simulink model "esc_motor_model_r2017a"  (R2017a)
settings: Solver=VariableStepAuto  StartTime=0.0  StopTime=20  RelTol=1e-3
settings Model: Creator=tdarrah  LastModifiedBy=tdarrah
settings SFSimCC: SimUseLocalCustomCode=on
settings RTWCC: RTWUseLocalCustomCode=on

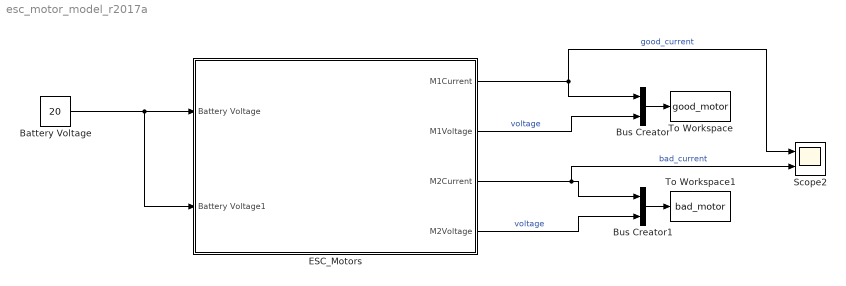
== system esc_motor_model_r2017a ==
  "Battery Voltage " : Constant  Value=20
  Bus Creator : BusCreator  Inputs=2
  Bus Creator1 : BusCreator  Inputs=2
  ESC_Motors : Subsystem
  Scope2 : Scope  NumInputPorts=2
  To Workspace : ToWorkspace  VariableName=good_motor  SaveFormat=Timeseries  SampleTime=-1
  To Workspace1 : ToWorkspace  VariableName=bad_motor  SaveFormat=Timeseries  SampleTime=-1
  wires:
  "Battery Voltage "/1 -> ESC_Motors/2(Battery Voltage1), ESC_Motors/1(Battery Voltage)
  ESC_Motors/1(M1Current) -> Scope2/1, Bus Creator/1  "good_current"
  ESC_Motors/2(M1Voltage) -> Bus Creator/2  "voltage"
  Bus Creator/1 -> To Workspace/1
  ESC_Motors/4(M2Voltage) -> Bus Creator1/2  "voltage"
  ESC_Motors/3(M2Current) -> Scope2/2, Bus Creator1/1  "bad_current"
  Bus Creator1/1 -> To Workspace1/1

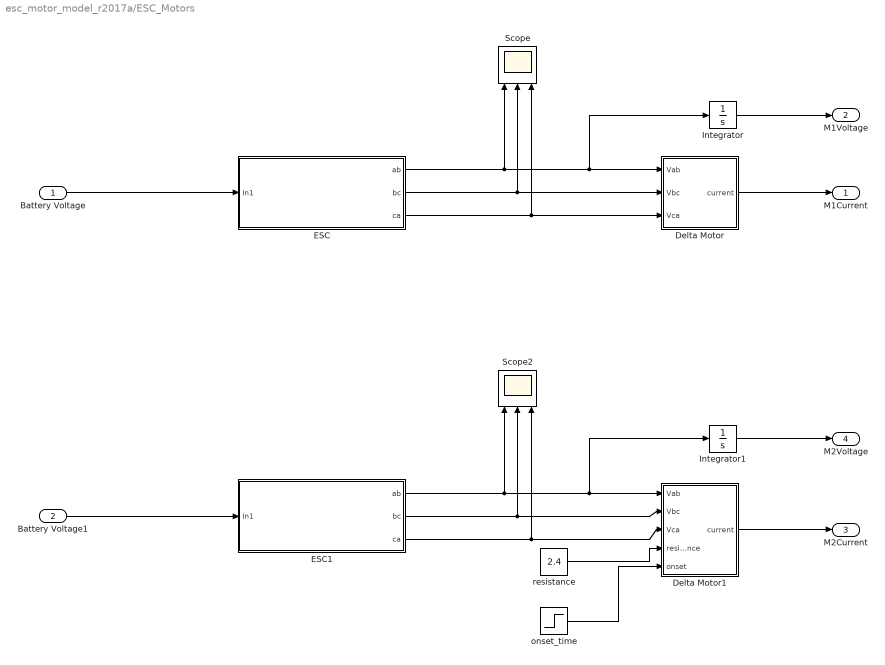
== system esc_motor_model_r2017a/ESC_Motors ==
  Battery Voltage : Inport
  Battery Voltage1 : Inport  Port=2
  Delta Motor : Subsystem
  Delta Motor1 : Subsystem
  ESC : Subsystem
  ESC1 : Subsystem
  Integrator : Integrator
  Integrator1 : Integrator
  Scope : Scope  NumInputPorts=3
  Scope2 : Scope  NumInputPorts=3
  "onset_time " : Step  Time=10  SampleTime=0
  resistance : Constant  Value=2.4
  M1Current : Outport
  M1Voltage : Outport  Port=2
  M2Current : Outport  Port=3
  M2Voltage : Outport  Port=4
  wires:
  Delta Motor/1(current) -> M1Current/1
  Integrator/1 -> M1Voltage/1
  ESC/2(bc) -> Scope/2, Delta Motor/2(Vbc)
  ESC/1(ab) -> Integrator/1, Delta Motor/1(Vab), Scope/1
  ESC/3(ca) -> Scope/3, Delta Motor/3(Vca)
  Battery Voltage/1 -> ESC/1(In1)
  Battery Voltage1/1 -> ESC1/1(In1)
  ESC1/1(ab) -> Integrator1/1, Delta Motor1/1(Vab), Scope2/1
  Delta Motor1/1(current) -> M2Current/1
  Integrator1/1 -> M2Voltage/1
  ESC1/3(ca) -> Scope2/3, Delta Motor1/3(Vca)
  ESC1/2(bc) -> Scope2/2, Delta Motor1/2(Vbc)
  resistance/1 -> Delta Motor1/4(resistance)
  "onset_time "/1 -> Delta Motor1/5(onset)

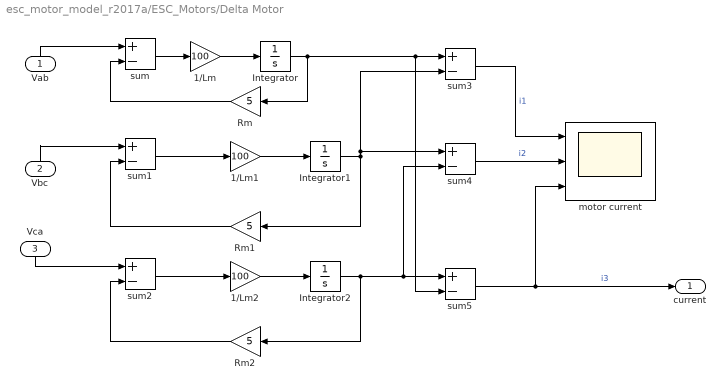
== system esc_motor_model_r2017a/ESC_Motors/Delta Motor ==
  Vab : Inport
  Vbc : Inport  Port=2
  Vca : Inport  Port=3
  1/Lm : Gain  Gain=100
  1/Lm1 : Gain  Gain=100
  1/Lm2 : Gain  Gain=100
  Integrator : Integrator
  Integrator1 : Integrator
  Integrator2 : Integrator
  Rm : Gain  Gain=5
  Rm1 : Gain  Gain=5
  Rm2 : Gain  Gain=5
  motor current : Scope  NumInputPorts=3
  sum{,1..5} (6 alike) : Sum  Inputs=+-
  current : Outport
  wires:
  1/Lm2/1 -> Integrator2/1
  Integrator/1 -> sum5/2, sum3/1, Rm/1
  sum3/1 -> motor current/1  "i1"
  Vab/1 -> sum/1
  Rm/1 -> sum/2
  Integrator1/1 -> sum4/1, sum3/2, Rm1/1
  sum1/1 -> 1/Lm1/1
  sum/1 -> 1/Lm/1
  1/Lm1/1 -> Integrator1/1
  Integrator2/1 -> sum5/1, sum4/2, Rm2/1
  1/Lm/1 -> Integrator/1
  sum4/1 -> motor current/2  "i2"
  Rm1/1 -> sum1/2
  Vca/1 -> sum2/1
  sum5/1 -> motor current/3, current/1  "i3"
  sum2/1 -> 1/Lm2/1
  Rm2/1 -> sum2/2
  Vbc/1 -> sum1/1

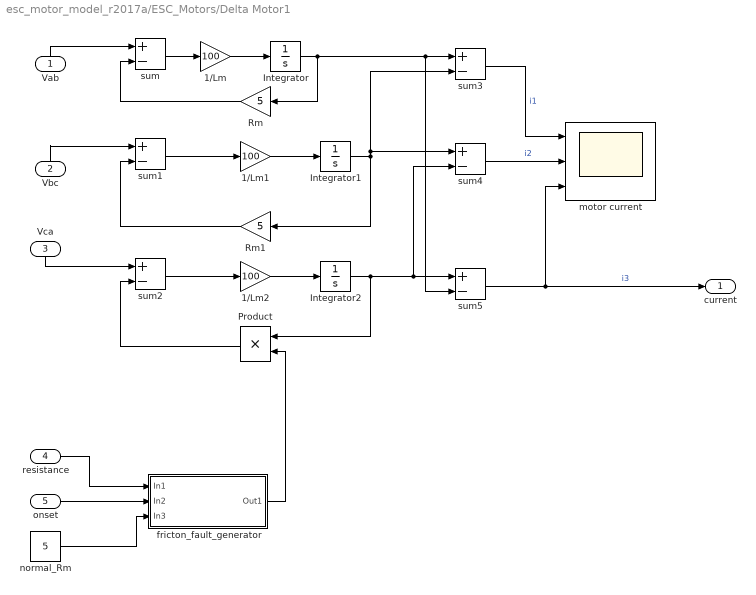
== system esc_motor_model_r2017a/ESC_Motors/Delta Motor1 ==
  Vab : Inport
  Vbc : Inport  Port=2
  Vca : Inport  Port=3
  resistance : Inport  Port=4
  onset : Inport  Port=5
  1/Lm : Gain  Gain=100
  1/Lm1 : Gain  Gain=100
  1/Lm2 : Gain  Gain=100
  Integrator : Integrator
  Integrator1 : Integrator
  Integrator2 : Integrator
  Product : Product
  Rm : Gain  Gain=5
  Rm1 : Gain  Gain=5
  fricton_fault_generator : Subsystem
  motor current : Scope  NumInputPorts=3
  normal_Rm : Constant  Value=5
  sum{,1..5} (6 alike) : Sum  Inputs=+-
  current : Outport
  wires:
  1/Lm2/1 -> Integrator2/1
  Integrator/1 -> sum5/2, sum3/1, Rm/1
  sum3/1 -> motor current/1  "i1"
  Vab/1 -> sum/1
  Rm/1 -> sum/2
  Integrator1/1 -> sum4/1, sum3/2, Rm1/1
  sum1/1 -> 1/Lm1/1
  sum/1 -> 1/Lm/1
  1/Lm1/1 -> Integrator1/1
  Integrator2/1 -> Product/1, sum5/1, sum4/2
  1/Lm/1 -> Integrator/1
  sum4/1 -> motor current/2  "i2"
  Rm1/1 -> sum1/2
  Vca/1 -> sum2/1
  sum5/1 -> motor current/3, current/1  "i3"
  sum2/1 -> 1/Lm2/1
  Product/1 -> sum2/2
  Vbc/1 -> sum1/1
  resistance/1 -> fricton_fault_generator/1(In1)
  onset/1 -> fricton_fault_generator/2(In2)
  normal_Rm/1 -> fricton_fault_generator/3(In3)
  fricton_fault_generator/1(Out1) -> Product/2

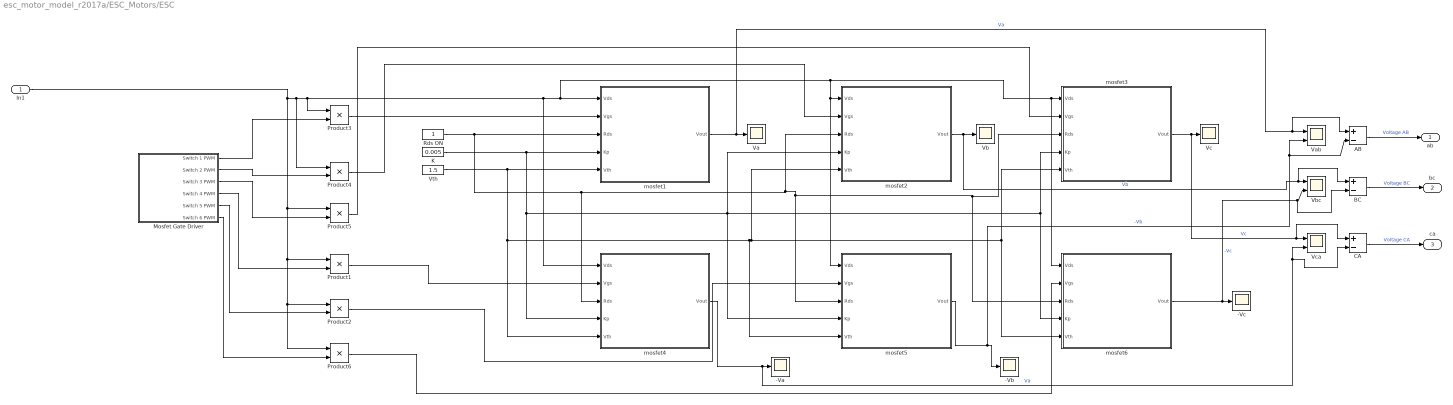
== system esc_motor_model_r2017a/ESC_Motors/ESC ==
  In1 : Inport
  -Va : Scope
  -Vb : Scope
  -Vc : Scope
  AB : Sum  Inputs=+-
  BC : Sum  Inputs=+-
  CA : Sum  Inputs=+-
  K : Constant  Value=0.005
  Mosfet Gate Driver : Subsystem
  Product{1..6} (6 alike) : Product
  Rds ON : Constant
  Va : Scope
  Vab : Scope  NumInputPorts=2
  Vb : Scope
  Vbc : Scope  NumInputPorts=2
  Vc : Scope
  Vca : Scope  NumInputPorts=2
  Vth : Constant  Value=1.5
  mosfet1 : MATLAB Function  TreatAsAtomicUnit=on
  mosfet2 : MATLAB Function  TreatAsAtomicUnit=on
  mosfet3 : MATLAB Function  TreatAsAtomicUnit=on
  mosfet4 : MATLAB Function  TreatAsAtomicUnit=on
  mosfet5 : MATLAB Function  TreatAsAtomicUnit=on
  mosfet6 : MATLAB Function  TreatAsAtomicUnit=on
  ab : Outport
  bc : Outport  Port=2
  ca : Outport  Port=3
  wires:
  mosfet2/1(Vout) -> BC/1, Vbc/1, Vb/1  "Vb"
  Mosfet Gate Driver/4(Switch 4 PWM) -> Product1/2
  CA/1 -> ca/1  "Voltage CA"
  Product5/1 -> mosfet3/2(Vgs)
  Mosfet Gate Driver/6(Switch 6 PWM) -> Product6/2
  BC/1 -> bc/1  "Voltage BC"
  Product2/1 -> mosfet5/2(Vgs)
  mosfet5/1(Vout) -> AB/2, Vab/2, -Vb/1  "-Vb"
  mosfet4/1(Vout) -> CA/2, Vca/2, -Va/1  "Va"
  Product4/1 -> mosfet2/2(Vgs)
  In1/1 -> Product6/1, Product2/1, Product1/1, Product5/1, Product4/1, mosfet4/1(Vds), mosfet6/1(Vds), mosfet3/1(Vds), mosfet5/1(Vds), mosfet2/1(Vds), mosfet1/1(Vds), Product3/1
  Mosfet Gate Driver/1(Switch 1 PWM) -> Product3/2
  mosfet6/1(Vout) -> BC/2, Vbc/2, -Vc/1  "-Vc"
  Product1/1 -> mosfet4/2(Vgs)
  AB/1 -> ab/1  "Voltage AB"
  Rds ON/1 -> mosfet1/3(Rds), mosfet4/3(Rds), mosfet3/3(Rds), mosfet6/3(Rds), mosfet5/3(Rds), mosfet2/3(Rds)
  Vth/1 -> mosfet4/5(Vth), mosfet5/5(Vth), mosfet2/5(Vth), mosfet6/5(Vth), mosfet3/5(Vth), mosfet1/5(Vth)
  mosfet3/1(Vout) -> CA/1, Vca/1, Vc/1  "Vc"
  Mosfet Gate Driver/2(Switch 2 PWM) -> Product4/2
  Mosfet Gate Driver/5(Switch 5 PWM) -> Product2/2
  Mosfet Gate Driver/3(Switch 3 PWM) -> Product5/2
  mosfet1/1(Vout) -> AB/1, Vab/1, Va/1  "Va"
  Product3/1 -> mosfet1/2(Vgs)
  K/1 -> mosfet4/4(Kp), mosfet5/4(Kp), mosfet2/4(Kp), mosfet6/4(Kp), mosfet3/4(Kp), mosfet1/4(Kp)
  Product6/1 -> mosfet6/2(Vgs)

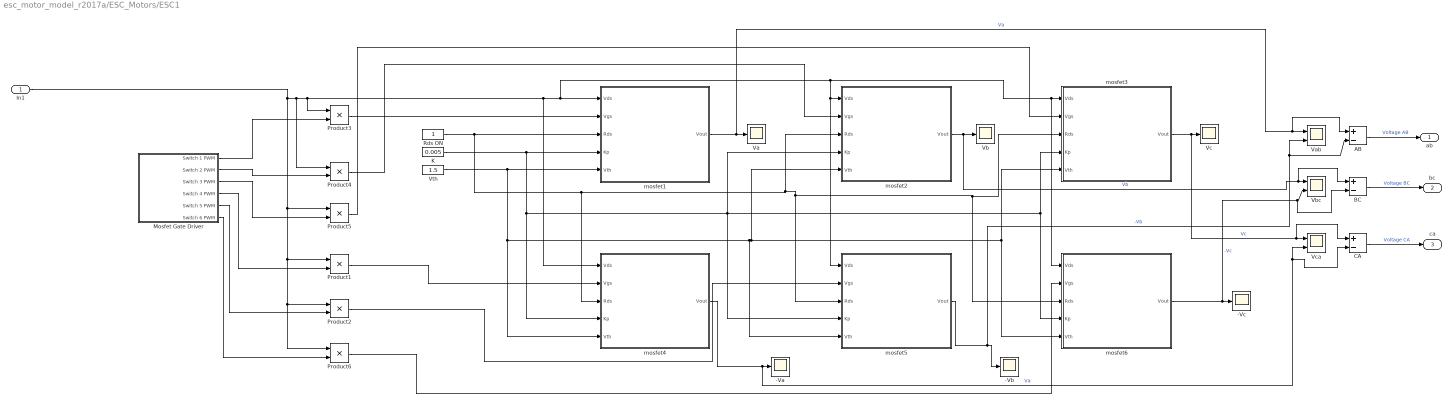
== system esc_motor_model_r2017a/ESC_Motors/ESC1 ==
  In1 : Inport
  -Va : Scope
  -Vb : Scope
  -Vc : Scope
  AB : Sum  Inputs=+-
  BC : Sum  Inputs=+-
  CA : Sum  Inputs=+-
  K : Constant  Value=0.005
  Mosfet Gate Driver : Subsystem
  Product{1..6} (6 alike) : Product
  Rds ON : Constant
  Va : Scope
  Vab : Scope  NumInputPorts=2
  Vb : Scope
  Vbc : Scope  NumInputPorts=2
  Vc : Scope
  Vca : Scope  NumInputPorts=2
  Vth : Constant  Value=1.5
  mosfet1 : MATLAB Function  TreatAsAtomicUnit=on
  mosfet2 : MATLAB Function  TreatAsAtomicUnit=on
  mosfet3 : MATLAB Function  TreatAsAtomicUnit=on
  mosfet4 : MATLAB Function  TreatAsAtomicUnit=on
  mosfet5 : MATLAB Function  TreatAsAtomicUnit=on
  mosfet6 : MATLAB Function  TreatAsAtomicUnit=on
  ab : Outport
  bc : Outport  Port=2
  ca : Outport  Port=3
  wires:
  mosfet2/1(Vout) -> BC/1, Vbc/1, Vb/1  "Vb"
  Mosfet Gate Driver/4(Switch 4 PWM) -> Product1/2
  CA/1 -> ca/1  "Voltage CA"
  Product5/1 -> mosfet3/2(Vgs)
  Mosfet Gate Driver/6(Switch 6 PWM) -> Product6/2
  BC/1 -> bc/1  "Voltage BC"
  Product2/1 -> mosfet5/2(Vgs)
  mosfet5/1(Vout) -> AB/2, Vab/2, -Vb/1  "-Vb"
  mosfet4/1(Vout) -> CA/2, Vca/2, -Va/1  "Va"
  Product4/1 -> mosfet2/2(Vgs)
  In1/1 -> Product6/1, Product2/1, Product1/1, Product5/1, Product4/1, mosfet4/1(Vds), mosfet6/1(Vds), mosfet3/1(Vds), mosfet5/1(Vds), mosfet2/1(Vds), mosfet1/1(Vds), Product3/1
  Mosfet Gate Driver/1(Switch 1 PWM) -> Product3/2
  mosfet6/1(Vout) -> BC/2, Vbc/2, -Vc/1  "-Vc"
  Product1/1 -> mosfet4/2(Vgs)
  AB/1 -> ab/1  "Voltage AB"
  Rds ON/1 -> mosfet1/3(Rds), mosfet4/3(Rds), mosfet3/3(Rds), mosfet6/3(Rds), mosfet5/3(Rds), mosfet2/3(Rds)
  Vth/1 -> mosfet4/5(Vth), mosfet5/5(Vth), mosfet2/5(Vth), mosfet6/5(Vth), mosfet3/5(Vth), mosfet1/5(Vth)
  mosfet3/1(Vout) -> CA/1, Vca/1, Vc/1  "Vc"
  Mosfet Gate Driver/2(Switch 2 PWM) -> Product4/2
  Mosfet Gate Driver/5(Switch 5 PWM) -> Product2/2
  Mosfet Gate Driver/3(Switch 3 PWM) -> Product5/2
  mosfet1/1(Vout) -> AB/1, Vab/1, Va/1  "Va"
  Product3/1 -> mosfet1/2(Vgs)
  K/1 -> mosfet4/4(Kp), mosfet5/4(Kp), mosfet2/4(Kp), mosfet6/4(Kp), mosfet3/4(Kp), mosfet1/4(Kp)
  Product6/1 -> mosfet6/2(Vgs)

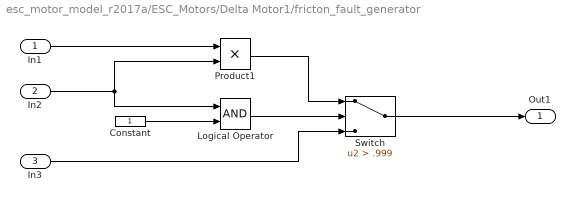
== system esc_motor_model_r2017a/ESC_Motors/Delta Motor1/fricton_fault_generator ==
  In1 : Inport
  In2 : Inport  Port=2
  In3 : Inport  Port=3
  Constant : Constant
  Logical Operator : Logic  AllPortsSameDT=off  OutDataTypeStr=boolean
  Product1 : Product
  Switch : Switch  Criteria=u2 > Threshold  Threshold=.999
  Out1 : Outport
  wires:
  In2/1 -> Logical Operator/1, Product1/2
  Constant/1 -> Logical Operator/2
  Logical Operator/1 -> Switch/2
  In3/1 -> Switch/3
  Product1/1 -> Switch/1
  Switch/1 -> Out1/1
  In1/1 -> Product1/1

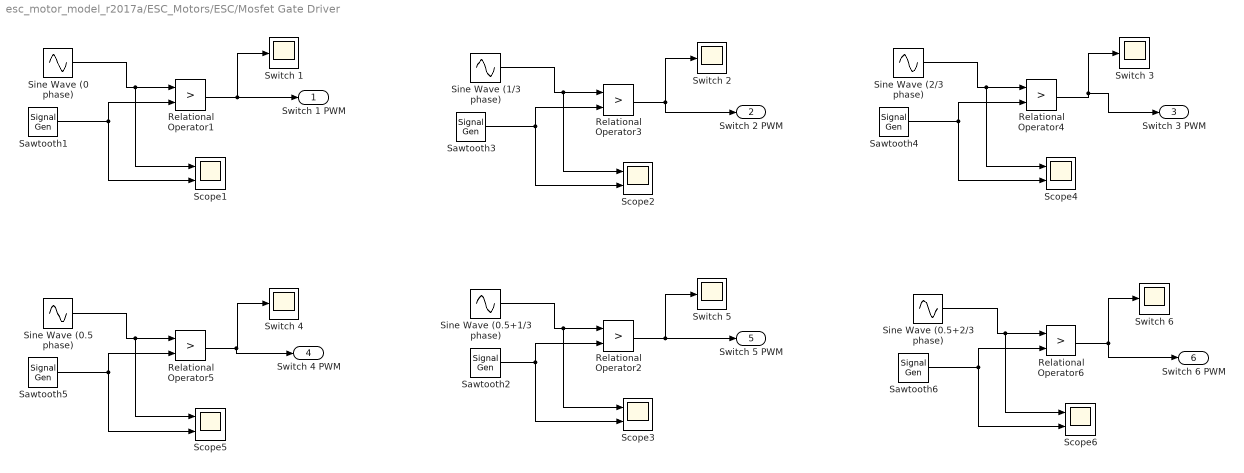
== system esc_motor_model_r2017a/ESC_Motors/ESC/Mosfet Gate Driver ==
  Relational Operator{1..6} (6 alike) : RelationalOperator  Operator=>  OutDataTypeStr=boolean  RndMeth=Simplest
  Sawtooth{1..6} (6 alike) : SignalGenerator  WaveForm=sawtooth  Frequency=20
  Scope{1..6} (6 alike) : Scope  NumInputPorts=2
  Sine Wave (0 phase) : Sin  Frequency=2*pi  SampleTime=0.001
  Sine Wave (0.5 phase) : Sin  Frequency=2*pi  Phase=0.5*(2*pi)  SampleTime=0.001
  Sine Wave (0.5+1/3 phase) : Sin  Frequency=2*pi  Phase=(0.5 + 1/3)*(2*pi)  SampleTime=0.001
  Sine Wave (0.5+2/3 phase) : Sin  Frequency=2*pi  Phase=(2/3 + 0.5)*2*pi  SampleTime=0.001
  Sine Wave (1/3 phase) : Sin  Frequency=2*pi  Phase=(1/3)*(2*pi)  SampleTime=0.001
  Sine Wave (2/3 phase) : Sin  Frequency=2*pi  Phase=(2/3)*(2*pi)  SampleTime=0.001
  Switch {1..6} (6 alike) : Scope
  Switch 1 PWM : Outport
  Switch 2 PWM : Outport  Port=2
  Switch 3 PWM : Outport  Port=3
  Switch 4 PWM : Outport  Port=4
  Switch 5 PWM : Outport  Port=5
  Switch 6 PWM : Outport  Port=6
  wires:
  Relational Operator4/1 -> Switch 3 PWM/1, Switch 3/1
  Sine Wave (1/3 phase)/1 -> Scope2/1, Relational Operator3/1
  Relational Operator6/1 -> Switch 6 PWM/1, Switch 6/1
  Sine Wave (2/3 phase)/1 -> Scope4/1, Relational Operator4/1
  Sawtooth4/1 -> Scope4/2, Relational Operator4/2
  Sawtooth1/1 -> Scope1/2, Relational Operator1/2
  Relational Operator2/1 -> Switch 5 PWM/1, Switch 5/1
  Sine Wave (0.5+2/3 phase)/1 -> Scope6/1, Relational Operator6/1
  Sawtooth5/1 -> Scope5/2, Relational Operator5/2
  Relational Operator1/1 -> Switch 1 PWM/1, Switch 1/1
  Sawtooth6/1 -> Scope6/2, Relational Operator6/2
  Sine Wave (0 phase)/1 -> Scope1/1, Relational Operator1/1
  Sine Wave (0.5 phase)/1 -> Scope5/1, Relational Operator5/1
  Relational Operator3/1 -> Switch 2 PWM/1, Switch 2/1
  Sine Wave (0.5+1/3 phase)/1 -> Scope3/1, Relational Operator2/1
  Sawtooth2/1 -> Scope3/2, Relational Operator2/2
  Sawtooth3/1 -> Scope2/2, Relational Operator3/2
  Relational Operator5/1 -> Switch 4 PWM/1, Switch 4/1

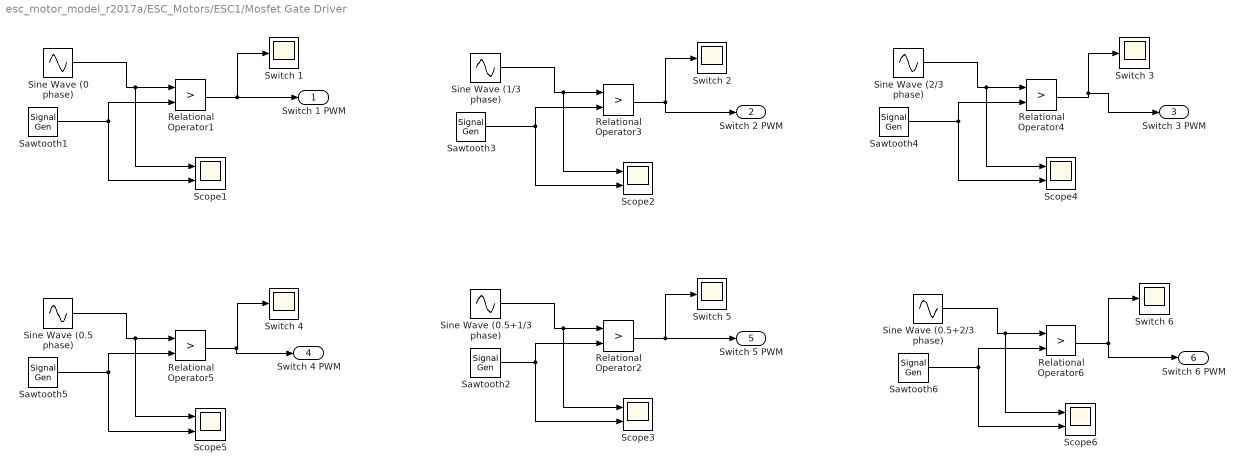
== system esc_motor_model_r2017a/ESC_Motors/ESC1/Mosfet Gate Driver ==
  Relational Operator{1..6} (6 alike) : RelationalOperator  Operator=>  OutDataTypeStr=boolean  RndMeth=Simplest
  Sawtooth{1..6} (6 alike) : SignalGenerator  WaveForm=sawtooth  Frequency=20
  Scope{1..6} (6 alike) : Scope  NumInputPorts=2
  Sine Wave (0 phase) : Sin  Frequency=2*pi  SampleTime=0.001
  Sine Wave (0.5 phase) : Sin  Frequency=2*pi  Phase=0.5*(2*pi)  SampleTime=0.001
  Sine Wave (0.5+1/3 phase) : Sin  Frequency=2*pi  Phase=(0.5 + 1/3)*(2*pi)  SampleTime=0.001
  Sine Wave (0.5+2/3 phase) : Sin  Frequency=2*pi  Phase=(2/3 + 0.5)*2*pi  SampleTime=0.001
  Sine Wave (1/3 phase) : Sin  Frequency=2*pi  Phase=(1/3)*(2*pi)  SampleTime=0.001
  Sine Wave (2/3 phase) : Sin  Frequency=2*pi  Phase=(2/3)*(2*pi)  SampleTime=0.001
  Switch {1..6} (6 alike) : Scope
  Switch 1 PWM : Outport
  Switch 2 PWM : Outport  Port=2
  Switch 3 PWM : Outport  Port=3
  Switch 4 PWM : Outport  Port=4
  Switch 5 PWM : Outport  Port=5
  Switch 6 PWM : Outport  Port=6
  wires:
  Relational Operator4/1 -> Switch 3 PWM/1, Switch 3/1
  Sine Wave (1/3 phase)/1 -> Scope2/1, Relational Operator3/1
  Relational Operator6/1 -> Switch 6 PWM/1, Switch 6/1
  Sine Wave (2/3 phase)/1 -> Scope4/1, Relational Operator4/1
  Sawtooth4/1 -> Scope4/2, Relational Operator4/2
  Sawtooth1/1 -> Scope1/2, Relational Operator1/2
  Relational Operator2/1 -> Switch 5 PWM/1, Switch 5/1
  Sine Wave (0.5+2/3 phase)/1 -> Scope6/1, Relational Operator6/1
  Sawtooth5/1 -> Scope5/2, Relational Operator5/2
  Relational Operator1/1 -> Switch 1 PWM/1, Switch 1/1
  Sawtooth6/1 -> Scope6/2, Relational Operator6/2
  Sine Wave (0 phase)/1 -> Scope1/1, Relational Operator1/1
  Sine Wave (0.5 phase)/1 -> Scope5/1, Relational Operator5/1
  Relational Operator3/1 -> Switch 2 PWM/1, Switch 2/1
  Sine Wave (0.5+1/3 phase)/1 -> Scope3/1, Relational Operator2/1
  Sawtooth2/1 -> Scope3/2, Relational Operator2/2
  Sawtooth3/1 -> Scope2/2, Relational Operator3/2
  Relational Operator5/1 -> Switch 4 PWM/1, Switch 4/1

== matlab function esc_motor_model_r2017a/ESC_Motors/ESC1/mosfet1 ==
  data: Vds input; Vgs input; Rds input; Kp input; Vth input; Vout output
function Vout   = MOSFET(Vds, Vgs, Rds, Kp, Vth)
% @input: 
%   Vds - source voltage
%   Vgs - gate voltage
%   Rds - drain source resistance
%   Kp - transconductance
%
% @output: output voltage
Ids = 0;
Vd = 0;
    % cutoff region
    if Vgs <= Vth
        Vd = 0;
        Ids = 0;
        
    % linear region  
    elseif Vds<(Vgs-Vth)
        Vd = Vds; 
        Ids = Kp*(((Vgs - Vth)*Vds)-((Vds^2)/2));
        
     % saturation region   
    elseif (Vgs-Vth)<Vds
         Vd = Vds;
         Ids = (Kp/2)*((Vgs-Vth)^2);         
    end

%calculate voltage output to the motor
Vout = Vd - Ids*Rds;

== matlab function esc_motor_model_r2017a/ESC_Motors/ESC/mosfet2 ==
  data: Vds input; Vgs input; Rds input; Kp input; Vth input; Vout output
function Vout   = MOSFET(Vds, Vgs, Rds, Kp, Vth)
% @input: 
%   Vds - source voltage
%   Vgs - gate voltage
%   Rds - drain source resistance
%   Kp - transconductance
%
% @output: output voltage
Ids = 0;
Vd = 0;
    % cutoff region
    if Vgs <= Vth
        Vd = 0;
        Ids = 0;
        
    % linear region  
    elseif Vds<(Vgs-Vth)
        Vd = Vds; 
        Ids = Kp*(((Vgs - Vth)*Vds)-((Vds^2)/2));
        
     % saturation region   
    elseif (Vgs-Vth)<Vds
         Vd = Vds;
         Ids = (Kp/2)*((Vgs-Vth)^2);         
    end

%calculate voltage output to the motor
Vout = Vd - Ids*Rds;

== matlab function esc_motor_model_r2017a/ESC_Motors/ESC/mosfet3 ==
  data: Vds input; Vgs input; Rds input; Kp input; Vth input; Vout output
function Vout   = MOSFET(Vds, Vgs, Rds, Kp, Vth)
% @input: 
%   Vds - source voltage
%   Vgs - gate voltage
%   Rds - drain source resistance
%   Kp - transconductance
%
% @output: output voltage
Ids = 0;
Vd = 0;
    % cutoff region
    if Vgs <= Vth
        Vd = 0;
        Ids = 0;
        
    % linear region  
    elseif Vds<(Vgs-Vth)
        Vd = Vds; 
        Ids = Kp*(((Vgs - Vth)*Vds)-((Vds^2)/2));
        
     % saturation region   
    elseif (Vgs-Vth)<Vds
         Vd = Vds;
         Ids = (Kp/2)*((Vgs-Vth)^2);         
    end

%calculate voltage output to the motor
Vout = Vd - Ids*Rds;

== matlab function esc_motor_model_r2017a/ESC_Motors/ESC/mosfet4 ==
  data: Vds input; Vgs input; Rds input; Kp input; Vth input; Vout output
function Vout   = MOSFET(Vds, Vgs, Rds, Kp, Vth)
% @input: 
%   Vds - source voltage
%   Vgs - gate voltage
%   Rds - drain source resistance
%   Kp - transconductance
%
% @output: output voltage
Ids = 0;
Vd = 0;
    % cutoff region
    if Vgs <= Vth
        Vd = 0;
        Ids = 0;
        
    % linear region  
    elseif Vds<(Vgs-Vth)
        Vd = Vds; 
        Ids = Kp*(((Vgs - Vth)*Vds)-((Vds^2)/2));
        
     % saturation region   
    elseif (Vgs-Vth)<Vds
         Vd = Vds;
         Ids = (Kp/2)*((Vgs-Vth)^2);         
    end

%calculate voltage output to the motor
Vout = Vd - Ids*Rds;

== matlab function esc_motor_model_r2017a/ESC_Motors/ESC/mosfet5 ==
  data: Vds input; Vgs input; Rds input; Kp input; Vth input; Vout output
function Vout   = MOSFET(Vds, Vgs, Rds, Kp, Vth)
% @input: 
%   Vds - source voltage
%   Vgs - gate voltage
%   Rds - drain source resistance
%   Kp - transconductance
%
% @output: output voltage
Ids = 0;
Vd = 0;
    % cutoff region
    if Vgs <= Vth
        Vd = 0;
        Ids = 0;
        
    % linear region  
    elseif Vds<(Vgs-Vth)
        Vd = Vds; 
        Ids = Kp*(((Vgs - Vth)*Vds)-((Vds^2)/2));
        
     % saturation region   
    elseif (Vgs-Vth)<Vds
         Vd = Vds;
         Ids = (Kp/2)*((Vgs-Vth)^2);         
    end

%calculate voltage output to the motor
Vout = Vd - Ids*Rds;

== matlab function esc_motor_model_r2017a/ESC_Motors/ESC/mosfet6 ==
  data: Vds input; Vgs input; Rds input; Kp input; Vth input; Vout output
function Vout   = MOSFET(Vds, Vgs, Rds, Kp, Vth)
% @input: 
%   Vds - source voltage
%   Vgs - gate voltage
%   Rds - drain source resistance
%   Kp - transconductance
%
% @output: output voltage
Ids = 0;
Vd = 0;
    % cutoff region
    if Vgs <= Vth
        Vd = 0;
        Ids = 0;
        
    % linear region  
    elseif Vds<(Vgs-Vth)
        Vd = Vds; 
        Ids = Kp*(((Vgs - Vth)*Vds)-((Vds^2)/2));
        
     % saturation region   
    elseif (Vgs-Vth)<Vds
         Vd = Vds;
         Ids = (Kp/2)*((Vgs-Vth)^2);         
    end

%calculate voltage output to the motor
Vout = Vd - Ids*Rds;

== matlab function esc_motor_model_r2017a/ESC_Motors/ESC1/mosfet2 ==
  data: Vds input; Vgs input; Rds input; Kp input; Vth input; Vout output
function Vout   = MOSFET(Vds, Vgs, Rds, Kp, Vth)
% @input: 
%   Vds - source voltage
%   Vgs - gate voltage
%   Rds - drain source resistance
%   Kp - transconductance
%
% @output: output voltage
Ids = 0;
Vd = 0;
    % cutoff region
    if Vgs <= Vth
        Vd = 0;
        Ids = 0;
        
    % linear region  
    elseif Vds<(Vgs-Vth)
        Vd = Vds; 
        Ids = Kp*(((Vgs - Vth)*Vds)-((Vds^2)/2));
        
     % saturation region   
    elseif (Vgs-Vth)<Vds
         Vd = Vds;
         Ids = (Kp/2)*((Vgs-Vth)^2);         
    end

%calculate voltage output to the motor
Vout = Vd - Ids*Rds;

== matlab function esc_motor_model_r2017a/ESC_Motors/ESC1/mosfet3 ==
  data: Vds input; Vgs input; Rds input; Kp input; Vth input; Vout output
function Vout   = MOSFET(Vds, Vgs, Rds, Kp, Vth)
% @input: 
%   Vds - source voltage
%   Vgs - gate voltage
%   Rds - drain source resistance
%   Kp - transconductance
%
% @output: output voltage
Ids = 0;
Vd = 0;
    % cutoff region
    if Vgs <= Vth
        Vd = 0;
        Ids = 0;
        
    % linear region  
    elseif Vds<(Vgs-Vth)
        Vd = Vds; 
        Ids = Kp*(((Vgs - Vth)*Vds)-((Vds^2)/2));
        
     % saturation region   
    elseif (Vgs-Vth)<Vds
         Vd = Vds;
         Ids = (Kp/2)*((Vgs-Vth)^2);         
    end

%calculate voltage output to the motor
Vout = Vd - Ids*Rds;

== matlab function esc_motor_model_r2017a/ESC_Motors/ESC/mosfet1 ==
  data: Vds input; Vgs input; Rds input; Kp input; Vth input; Vout output
function Vout   = MOSFET(Vds, Vgs, Rds, Kp, Vth)
% @input: 
%   Vds - source voltage
%   Vgs - gate voltage
%   Rds - drain source resistance
%   Kp - transconductance
%
% @output: output voltage
Ids = 0;
Vd = 0;
    % cutoff region
    if Vgs <= Vth
        Vd = 0;
        Ids = 0;
        
    % linear region  
    elseif Vds<(Vgs-Vth)
        Vd = Vds; 
        Ids = Kp*(((Vgs - Vth)*Vds)-((Vds^2)/2));
        
     % saturation region   
    elseif (Vgs-Vth)<Vds
         Vd = Vds;
         Ids = (Kp/2)*((Vgs-Vth)^2);         
    end

%calculate voltage output to the motor
Vout = Vd - Ids*Rds;

== matlab function esc_motor_model_r2017a/ESC_Motors/ESC1/mosfet4 ==
  data: Vds input; Vgs input; Rds input; Kp input; Vth input; Vout output
function Vout   = MOSFET(Vds, Vgs, Rds, Kp, Vth)
% @input: 
%   Vds - source voltage
%   Vgs - gate voltage
%   Rds - drain source resistance
%   Kp - transconductance
%
% @output: output voltage
Ids = 0;
Vd = 0;
    % cutoff region
    if Vgs <= Vth
        Vd = 0;
        Ids = 0;
        
    % linear region  
    elseif Vds<(Vgs-Vth)
        Vd = Vds; 
        Ids = Kp*(((Vgs - Vth)*Vds)-((Vds^2)/2));
        
     % saturation region   
    elseif (Vgs-Vth)<Vds
         Vd = Vds;
         Ids = (Kp/2)*((Vgs-Vth)^2);         
    end

%calculate voltage output to the motor
Vout = Vd - Ids*Rds;

== matlab function esc_motor_model_r2017a/ESC_Motors/ESC1/mosfet5 ==
  data: Vds input; Vgs input; Rds input; Kp input; Vth input; Vout output
function Vout   = MOSFET(Vds, Vgs, Rds, Kp, Vth)
% @input: 
%   Vds - source voltage
%   Vgs - gate voltage
%   Rds - drain source resistance
%   Kp - transconductance
%
% @output: output voltage
Ids = 0;
Vd = 0;
    % cutoff region
    if Vgs <= Vth
        Vd = 0;
        Ids = 0;
        
    % linear region  
    elseif Vds<(Vgs-Vth)
        Vd = Vds; 
        Ids = Kp*(((Vgs - Vth)*Vds)-((Vds^2)/2));
        
     % saturation region   
    elseif (Vgs-Vth)<Vds
         Vd = Vds;
         Ids = (Kp/2)*((Vgs-Vth)^2);         
    end

%calculate voltage output to the motor
Vout = Vd - Ids*Rds;

== matlab function esc_motor_model_r2017a/ESC_Motors/ESC1/mosfet6 ==
  data: Vds input; Vgs input; Rds input; Kp input; Vth input; Vout output
function Vout   = MOSFET(Vds, Vgs, Rds, Kp, Vth)
% @input: 
%   Vds - source voltage
%   Vgs - gate voltage
%   Rds - drain source resistance
%   Kp - transconductance
%
% @output: output voltage
Ids = 0;
Vd = 0;
    % cutoff region
    if Vgs <= Vth
        Vd = 0;
        Ids = 0;
        
    % linear region  
    elseif Vds<(Vgs-Vth)
        Vd = Vds; 
        Ids = Kp*(((Vgs - Vth)*Vds)-((Vds^2)/2));
        
     % saturation region   
    elseif (Vgs-Vth)<Vds
         Vd = Vds;
         Ids = (Kp/2)*((Vgs-Vth)^2);         
    end

%calculate voltage output to the motor
Vout = Vd - Ids*Rds;
